simulink model "Requirements_Table"  (R2022b)
settings: Solver=FixedStepAuto  StartTime=0.0  StopTime=10.0  FixedStep=1e-3  RelTol=1e-3  EnableMultiTasking=on
settings Model: ExtModeTrigDuration=5  Creator=Ali Umar  LastModifiedBy=Ali Umar
settings OptimizationCC: EnhancedBackFolding=on  PassReuseOutputArgsAs=Individual arguments  ZeroExternalMemoryAtStartup=off  ZeroInternalMemoryAtStartup=off  MaxStackSize=64  OptimizeBlockOrder=speed  DifferentSizesBufferReuse=on  OptimizationCustomize=off  EfficientTunableParamExpr=on
settings DebuggingCC: ParameterTunabilityLossMsg=error
settings HardwareCC: ProdBitPerPointer=32  ProdBitPerSizeT=32  ProdBitPerPtrDiffT=32  ProdLargestAtomicInteger=Long  ProdLargestAtomicFloat=Double  ProdWordSize=32  ProdHWDeviceType=ARM Compatible->ARM Cortex
settings SFSimCC: MATLABDynamicMemAlloc=off
settings RTWCC: Description=Embedded Coder  SystemTargetFile=ert.tlc  HardwareBoard=NXP FRDM-K64F  TLCOptions="-aInlineSetEventsForThisBaseRateFcn=TLC_FALSE -aSuppressMultiTaskScheduler=TLC_FALSE  -aRateBasedStepFcn=0"  TemplateMakefile=ert_default_tmf  Toolchain=GNU Tools for ARM Embedded Processors
settings CodeAppCC: ForceParamTrailComments=on  IgnoreCustomStorageClasses=off  OperatorAnnotations=on  SimulinkDataObjDesc=on  SFDataObjDesc=on  InsertBlockDesc=on
settings ERTTargetCC: ExtModeTransport=4  ExtModeMexFile=sendToCommService

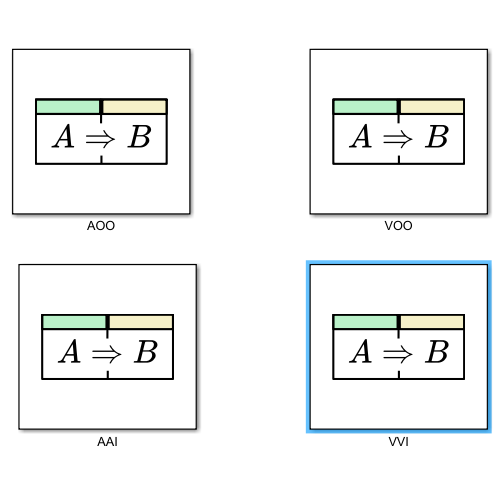
[thumbnail: Simulink's stored preview of the top-level diagram]
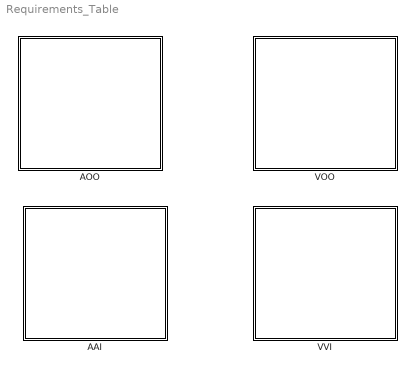
== system Requirements_Table ==
  AAI : Requirements Table  TreatAsAtomicUnit=on
  AOO : Requirements Table  TreatAsAtomicUnit=on
  VOO : Requirements Table  TreatAsAtomicUnit=on
  VVI : Requirements Table  TreatAsAtomicUnit=on

== stateflow chart Requirements_Table/VOO ==
  (default) -> (junction 1073741860)
  (junction 1073741860) -> (junction 1073741861) : {
      | % SF_REQ_REV_07
      | }
  (junction 1073741861) -> (junction 1073741863) : {
      | % HEADER_ASSIGNMENTS
      |
      | }
  (junction 1073741863) -> (junction 1073741865) : {
      | % START_A_4
      | }
  (junction 1073741865) -> (junction 1073741867) : {
      | }
  (junction 1073741867) -> (junction 1073741869)
  (junction 1073741869) -> (junction 1073741871) : {
      | }
  (junction 1073741871) -> (junction 1073741873) : {
      | % END_A_4
      | }
  (junction 1073741873) -> (junction 1073741976) : {
      | % START_R_1
      | }
  (junction 1073741976) -> (junction 1073741978) : {
      | }
  (junction 1073741978) -> (junction 1073741980)
  (junction 1073741980) -> (junction 1073741982) [order 1] : [duration((((ATR_PACE_CTRL) == (0))) && (((VENT_PACE_CTRL) == (1))) && (((PACE_CHARGE_CTRL) == (0))) && (((ATR_GND_CTRL) == (0))) && (((VENT_GND_CTRL) == (0)))) >= VPW]
  (junction 1073741980) -> (junction 1073741988) [order 2]
  (junction 1073741982) -> (junction 1073741984) : {
      | reqtable_postcondition((((ATR_PACE_CTRL) == (0))) && (((VENT_PACE_CTRL) == (0))) && (((PACING_REF_PWM) == (VA))) && (((PACE_CHARGE_CTRL) == (1))) && (((PACE_GND_CTRL) == (1))) && (((ATR_GND_CTRL) == (0))) && (((VENT_GND_CTRL) == (1))), 'R:1');
      | Charging C22 and Discharging C21
      |
      | }
  (junction 1073741984) -> (junction 1073741986) : {
      | }
  (junction 1073741986) -> (junction 1073741988)
  (junction 1073741988) -> (junction 1073741990)
  (junction 1073741990) -> (junction 1073741992) : {
      | % END_R_1
      | }
  (junction 1073741992) -> (junction 1073741955) : {
      | % START_R_7
      | }
  (junction 1073741955) -> (junction 1073741957) : {
      | }
  (junction 1073741957) -> (junction 1073741959)
  (junction 1073741959) -> (junction 1073741961) [order 1] : [duration((((ATR_PACE_CTRL) == (0))) && (((VENT_PACE_CTRL) == (0))) && (((PACING_REF_PWM) == (VA))) && (((PACE_CHARGE_CTRL) == (1))) && (((PACE_GND_CTRL) == (1))) && (((ATR_GND_CTRL) == (0))) && (((VENT_GND_CTRL) == (1)))) >= (60000/LRL)-VPW]
  (junction 1073741959) -> (junction 1073741967) [order 2]
  (junction 1073741961) -> (junction 1073741963) : {
      | reqtable_postcondition((((ATR_PACE_CTRL) == (0))) && (((VENT_PACE_CTRL) == (1))) && (((PACE_CHARGE_CTRL) == (0))) && (((ATR_GND_CTRL) == (0))) && (((VENT_GND_CTRL) == (0))), 'R:2');
      | VOO Pacing
      |
      | }
  (junction 1073741963) -> (junction 1073741965) : {
      | }
  (junction 1073741965) -> (junction 1073741967)
  (junction 1073741967) -> (junction 1073741969)
  (junction 1073741969) -> (junction 1073741971) : {
      | % END_R_7
      | }

== stateflow chart Requirements_Table/AAI ==
  (default) -> (junction 1073741860)
  (junction 1073741860) -> (junction 1073741861) : {
      | % SF_REQ_REV_07
      | }
  (junction 1073741861) -> (junction 1073741863) : {
      | % HEADER_ASSIGNMENTS
      |
      | }
  (junction 1073741863) -> (junction 1073741865) : {
      | % START_A_4
      | }
  (junction 1073741865) -> (junction 1073741867) : {
      | }
  (junction 1073741867) -> (junction 1073741869)
  (junction 1073741869) -> (junction 1073741871) : {
      | }
  (junction 1073741871) -> (junction 1073741873) : {
      | % END_A_4
      | }
  (junction 1073741873) -> (junction 1073742161) : {
      | % START_R_1
      | }
  (junction 1073742161) -> (junction 1073742163) : {
      | }
  (junction 1073742163) -> (junction 1073742165) : {
      | reqtable_postcondition((((FRONTEND_CTRL) == (1))) && (((ATR_CMP_REF_PWM) == (75))) && (((ATR_PACE_CTRL) == (0))) && (((VENT_PACE_CTRL) == (0))) && (((PACING_REF_PWM) == (75))) && (((PACE_CHARGE_CTRL) == (1))) && (((PACE_GND_CTRL) == (1))) && (((VENT_PACE_CTRL) == (0))) && (((ATR_PACE_CTRL) == (0))) && (((VENT_GND_CTRL) == (0))) && (((ATR_GND_CTRL) == (1))), 'R:1');
      | Startup Action
      |
      | }
  (junction 1073742165) -> (junction 1073742167) : {
      | }
  (junction 1073742167) -> (junction 1073741951) : {
      | % END_R_1
      | }
  (junction 1073741951) -> (junction 1073742194) : {
      | % START_R_22
      | }
  (junction 1073742194) -> (junction 1073742196) : {
      | }
  (junction 1073742196) -> (junction 1073742198)
  (junction 1073742198) -> (junction 1073742200) [order 1] : [duration((((FRONTEND_CTRL) == (1))) && (((ATR_CMP_REF_PWM) == (75))) && (((ATR_CMP_DETECT) == (0))) && (((ATR_PACE_CTRL) == (0))) && (((VENT_PACE_CTRL) == (0))) && (((PACING_REF_PWM) == (75))) && (((PACE_CHARGE_CTRL) == (1))) && (((PACE_GND_CTRL) == (1))) && (((VENT_PACE_CTRL) == (0))) && (((ATR_PACE_CTRL) == (0))) && (((VENT_GND_CTRL) == (0))) && (((ATR_GND_CTRL) == (1)))) >= LRI]
  (junction 1073742198) -> (junction 1073742206) [order 2]
  (junction 1073742200) -> (junction 1073742202) : {
      | reqtable_postcondition((((PACE_CHARGE_CTRL) == (0))) && (((PACE_GND_CTRL) == (1))) && (((VENT_PACE_CTRL) == (0))) && (((ATR_PACE_CTRL) == (1))) && (((VENT_GND_CTRL) == (0))) && (((ATR_GND_CTRL) == (0))), 'R:2');
      | pacing from the start
      |
      | }
  (junction 1073742202) -> (junction 1073742204) : {
      | }
  (junction 1073742204) -> (junction 1073742206)
  (junction 1073742206) -> (junction 1073742208)
  (junction 1073742208) -> (junction 1073742210) : {
      | % END_R_22
      | }
  (junction 1073742210) -> (junction 1073742173) : {
      | % START_R_16
      | }
  (junction 1073742173) -> (junction 1073742175) : {
      | }
  (junction 1073742175) -> (junction 1073742177)
  (junction 1073742177) -> (junction 1073742179) [order 1] : [duration((((FRONTEND_CTRL) == (1))) && (((ATR_CMP_REF_PWM) == (75))) && (((ATR_CMP_DETECT) == (0)))) >= LRI-R]
  (junction 1073742177) -> (junction 1073742185) [order 2]
  (junction 1073742179) -> (junction 1073742181) : {
      | reqtable_postcondition((((PACE_CHARGE_CTRL) == (0))) && (((PACE_GND_CTRL) == (1))) && (((VENT_PACE_CTRL) == (0))) && (((ATR_PACE_CTRL) == (1))) && (((VENT_GND_CTRL) == (0))) && (((ATR_GND_CTRL) == (0))), 'R:3');
      | Pacing
      |
      | }
  (junction 1073742181) -> (junction 1073742183) : {
      | }
  (junction 1073742183) -> (junction 1073742185)
  (junction 1073742185) -> (junction 1073742187)
  (junction 1073742187) -> (junction 1073742189) : {
      | % END_R_16
      | }
  (junction 1073742189) -> (junction 1073741967) : {
      | % START_R_10
      | }
  (junction 1073741967) -> (junction 1073741969) : {
      | }
  (junction 1073741969) -> (junction 1073741971)
  (junction 1073741971) -> (junction 1073741973) [order 1] : [duration((((FRONTEND_CTRL) == (1))) && (((ATR_CMP_REF_PWM) == (75))) && (((ATR_CMP_DETECT) == (1))) && (((ATR_PACE_CTRL) == (0))) && (((VENT_PACE_CTRL) == (0))) && (((PACING_REF_PWM) == (75))) && (((PACE_CHARGE_CTRL) == (1))) && (((PACE_GND_CTRL) == (1))) && (((VENT_PACE_CTRL) == (0))) && (((ATR_PACE_CTRL) == (0))) && (((VENT_GND_CTRL) == (0))) && (((ATR_GND_CTRL) == (1)))) >= LRI]
  (junction 1073741971) -> (junction 1073741979) [order 2]
  (junction 1073741973) -> (junction 1073741975) : {
      | reqtable_postcondition((((ATR_PACE_CTRL) == (0))) && (((VENT_PACE_CTRL) == (0))) && (((PACING_REF_PWM) == (75))) && (((PACE_CHARGE_CTRL) == (1))) && (((PACE_GND_CTRL) == (1))) && (((VENT_PACE_CTRL) == (0))) && (((ATR_PACE_CTRL) == (0))) && (((VENT_GND_CTRL) == (0))) && (((ATR_GND_CTRL) == (1))), 'R:4');
      | Timer checks refractory period and chargs C22/ Discharges C21
      |
      | }
  (junction 1073741975) -> (junction 1073741977) : {
      | }
  (junction 1073741977) -> (junction 1073741979)
  (junction 1073741979) -> (junction 1073741981)
  (junction 1073741981) -> (junction 1073741983) : {
      | % END_R_10
      | }
  (junction 1073741983) -> (junction 1073742000) : {
      | % START_R_13
      | }
  (junction 1073742000) -> (junction 1073742002) : {
      | }
  (junction 1073742002) -> (junction 1073742004)
  (junction 1073742004) -> (junction 1073742006) [order 1] : [duration((((ATR_CMP_DETECT) == (0))) && (((ATR_PACE_CTRL) == (0))) && (((VENT_PACE_CTRL) == (0))) && (((PACING_REF_PWM) == (75))) && (((PACE_CHARGE_CTRL) == (1))) && (((PACE_GND_CTRL) == (1))) && (((VENT_PACE_CTRL) == (0))) && (((ATR_PACE_CTRL) == (0))) && (((VENT_GND_CTRL) == (0))) && (((ATR_GND_CTRL) == (1)))) >= R]
  (junction 1073742004) -> (junction 1073742012) [order 2]
  (junction 1073742006) -> (junction 1073742008) : {
      | reqtable_postcondition((((FRONTEND_CTRL) == (1))) && (((ATR_CMP_REF_PWM) == (75))), 'R:5');
      | Turns sensing on
      |
      | }
  (junction 1073742008) -> (junction 1073742010) : {
      | }
  (junction 1073742010) -> (junction 1073742012)
  (junction 1073742012) -> (junction 1073742014)
  (junction 1073742014) -> (junction 1073742101) : {
      | % END_R_13
      | }

== stateflow chart Requirements_Table/AOO ==
  (default) -> (junction 1073741860)
  (junction 1073741860) -> (junction 1073741861) : {
      | % SF_REQ_REV_07
      | }
  (junction 1073741861) -> (junction 1073741863) : {
      | % HEADER_ASSIGNMENTS
      |
      | }
  (junction 1073741863) -> (junction 1073741865) : {
      | % START_A_4
      | }
  (junction 1073741865) -> (junction 1073741867) : {
      | }
  (junction 1073741867) -> (junction 1073741869)
  (junction 1073741869) -> (junction 1073741871) : {
      | }
  (junction 1073741871) -> (junction 1073741873) : {
      | % END_A_4
      | }
  (junction 1073741873) -> (junction 1073741996) : {
      | % START_R_1
      | }
  (junction 1073741996) -> (junction 1073741998) : {
      | }
  (junction 1073741998) -> (junction 1073742000)
  (junction 1073742000) -> (junction 1073742002) [order 1] : [duration((((ATR_PACE_CTRL) == (1))) && (((VENT_PACE_CTRL) == (0))) && (((PACE_CHARGE_CTRL) == (0))) && (((ATR_GND_CTRL) == (0))) && (((VENT_GND_CTRL) == (0)))) >= APW]
  (junction 1073742000) -> (junction 1073742008) [order 2]
  (junction 1073742002) -> (junction 1073742004) : {
      | reqtable_postcondition((((ATR_PACE_CTRL) == (0))) && (((VENT_PACE_CTRL) == (0))) && (((PACING_REF_PWM) == (AA))) && (((PACE_CHARGE_CTRL) == (1))) && (((PACE_GND_CTRL) == (1))) && (((ATR_GND_CTRL) == (1))) && (((VENT_GND_CTRL) == (0))), 'R:1');
      | Charges C22 Capacitor
      |
      | }
  (junction 1073742004) -> (junction 1073742006) : {
      | }
  (junction 1073742006) -> (junction 1073742008)
  (junction 1073742008) -> (junction 1073742010)
  (junction 1073742010) -> (junction 1073742012) : {
      | % END_R_1
      | }
  (junction 1073742012) -> (junction 1073742017) : {
      | % START_R_10
      | }
  (junction 1073742017) -> (junction 1073742019) : {
      | }
  (junction 1073742019) -> (junction 1073742021)
  (junction 1073742021) -> (junction 1073742023) [order 1] : [duration((((ATR_PACE_CTRL) == (0))) && (((VENT_PACE_CTRL) == (0))) && (((PACING_REF_PWM) == (AA))) && (((PACE_CHARGE_CTRL) == (1))) && (((PACE_GND_CTRL) == (1))) && (((ATR_GND_CTRL) == (1))) && (((VENT_GND_CTRL) == (0)))) >= (60000/LRL)-APW]
  (junction 1073742021) -> (junction 1073742029) [order 2]
  (junction 1073742023) -> (junction 1073742025) : {
      | reqtable_postcondition((((ATR_PACE_CTRL) == (1))) && (((VENT_PACE_CTRL) == (0))) && (((PACE_CHARGE_CTRL) == (0))) && (((ATR_GND_CTRL) == (0))) && (((VENT_GND_CTRL) == (0))), 'R:2');
      | AOO pacing
      |
      | }
  (junction 1073742025) -> (junction 1073742027) : {
      | }
  (junction 1073742027) -> (junction 1073742029)
  (junction 1073742029) -> (junction 1073742031)
  (junction 1073742031) -> (junction 1073742033) : {
      | % END_R_10
      | }

== stateflow chart Requirements_Table/VVI ==
  (default) -> (junction 1073741860)
  (junction 1073741860) -> (junction 1073741861) : {
      | % SF_REQ_REV_07
      | }
  (junction 1073741861) -> (junction 1073741863) : {
      | % HEADER_ASSIGNMENTS
      |
      | }
  (junction 1073741863) -> (junction 1073741865) : {
      | % START_A_4
      | }
  (junction 1073741865) -> (junction 1073741867) : {
      | }
  (junction 1073741867) -> (junction 1073741869)
  (junction 1073741869) -> (junction 1073741871) : {
      | }
  (junction 1073741871) -> (junction 1073741873) : {
      | % END_A_4
      | }
  (junction 1073741873) -> (junction 1073742161) : {
      | % START_R_1
      | }
  (junction 1073742161) -> (junction 1073742163) : {
      | }
  (junction 1073742163) -> (junction 1073742165) : {
      | reqtable_postcondition((((FRONTEND_CTRL) == (1))) && (((ATR_CMP_REF_PWM) == (75))) && (((ATR_PACE_CTRL) == (0))) && (((VENT_PACE_CTRL) == (0))) && (((PACING_REF_PWM) == (75))) && (((PACE_CHARGE_CTRL) == (1))) && (((PACE_GND_CTRL) == (1))) && (((VENT_PACE_CTRL) == (0))) && (((ATR_PACE_CTRL) == (0))) && (((VENT_GND_CTRL) == (1))) && (((ATR_GND_CTRL) == (0))), 'R:1');
      | Startup Action
      |
      | }
  (junction 1073742165) -> (junction 1073742167) : {
      | }
  (junction 1073742167) -> (junction 1073741951) : {
      | % END_R_1
      | }
  (junction 1073741951) -> (junction 1073742194) : {
      | % START_R_22
      | }
  (junction 1073742194) -> (junction 1073742196) : {
      | }
  (junction 1073742196) -> (junction 1073742198)
  (junction 1073742198) -> (junction 1073742200) [order 1] : [duration((((FRONTEND_CTRL) == (1))) && (((ATR_CMP_REF_PWM) == (75))) && (((ATR_CMP_DETECT) == (0))) && (((ATR_PACE_CTRL) == (0))) && (((VENT_PACE_CTRL) == (0))) && (((PACING_REF_PWM) == (75))) && (((PACE_CHARGE_CTRL) == (1))) && (((PACE_GND_CTRL) == (1))) && (((VENT_PACE_CTRL) == (0))) && (((ATR_PACE_CTRL) == (0))) && (((VENT_GND_CTRL) == (1))) && (((ATR_GND_CTRL) == (0)))) >= LRI]
  (junction 1073742198) -> (junction 1073742206) [order 2]
  (junction 1073742200) -> (junction 1073742202) : {
      | reqtable_postcondition((((PACE_CHARGE_CTRL) == (0))) && (((PACE_GND_CTRL) == (1))) && (((VENT_PACE_CTRL) == (1))) && (((ATR_PACE_CTRL) == (0))) && (((VENT_GND_CTRL) == (0))) && (((ATR_GND_CTRL) == (0))), 'R:2');
      | pacing from the start
      |
      | }
  (junction 1073742202) -> (junction 1073742204) : {
      | }
  (junction 1073742204) -> (junction 1073742206)
  (junction 1073742206) -> (junction 1073742208)
  (junction 1073742208) -> (junction 1073742210) : {
      | % END_R_22
      | }
  (junction 1073742210) -> (junction 1073742173) : {
      | % START_R_16
      | }
  (junction 1073742173) -> (junction 1073742175) : {
      | }
  (junction 1073742175) -> (junction 1073742177)
  (junction 1073742177) -> (junction 1073742179) [order 1] : [duration((((FRONTEND_CTRL) == (1))) && (((ATR_CMP_REF_PWM) == (75))) && (((ATR_CMP_DETECT) == (0)))) >= LRI-R]
  (junction 1073742177) -> (junction 1073742185) [order 2]
  (junction 1073742179) -> (junction 1073742181) : {
      | reqtable_postcondition((((PACE_CHARGE_CTRL) == (0))) && (((PACE_GND_CTRL) == (1))) && (((VENT_PACE_CTRL) == (1))) && (((ATR_PACE_CTRL) == (0))) && (((VENT_GND_CTRL) == (0))) && (((ATR_GND_CTRL) == (0))), 'R:3');
      | Pacing
      |
      | }
  (junction 1073742181) -> (junction 1073742183) : {
      | }
  (junction 1073742183) -> (junction 1073742185)
  (junction 1073742185) -> (junction 1073742187)
  (junction 1073742187) -> (junction 1073742189) : {
      | % END_R_16
      | }
  (junction 1073742189) -> (junction 1073741967) : {
      | % START_R_10
      | }
  (junction 1073741967) -> (junction 1073741969) : {
      | }
  (junction 1073741969) -> (junction 1073741971)
  (junction 1073741971) -> (junction 1073741973) [order 1] : [duration((((FRONTEND_CTRL) == (1))) && (((ATR_CMP_REF_PWM) == (75))) && (((ATR_CMP_DETECT) == (1))) && (((ATR_PACE_CTRL) == (0))) && (((VENT_PACE_CTRL) == (0))) && (((PACING_REF_PWM) == (75))) && (((PACE_CHARGE_CTRL) == (1))) && (((PACE_GND_CTRL) == (1))) && (((VENT_PACE_CTRL) == (0))) && (((ATR_PACE_CTRL) == (0))) && (((VENT_GND_CTRL) == (1))) && (((ATR_GND_CTRL) == (0)))) >= LRI]
  (junction 1073741971) -> (junction 1073741979) [order 2]
  (junction 1073741973) -> (junction 1073741975) : {
      | reqtable_postcondition((((ATR_PACE_CTRL) == (0))) && (((VENT_PACE_CTRL) == (0))) && (((PACING_REF_PWM) == (75))) && (((PACE_CHARGE_CTRL) == (1))) && (((PACE_GND_CTRL) == (1))) && (((VENT_PACE_CTRL) == (0))) && (((ATR_PACE_CTRL) == (0))) && (((VENT_GND_CTRL) == (1))) && (((ATR_GND_CTRL) == (0))), 'R:4');
      | Timer checks refractory period and chargs C22/ Discharges C21
      |
      | }
  (junction 1073741975) -> (junction 1073741977) : {
      | }
  (junction 1073741977) -> (junction 1073741979)
  (junction 1073741979) -> (junction 1073741981)
  (junction 1073741981) -> (junction 1073741983) : {
      | % END_R_10
      | }
  (junction 1073741983) -> (junction 1073742000) : {
      | % START_R_13
      | }
  (junction 1073742000) -> (junction 1073742002) : {
      | }
  (junction 1073742002) -> (junction 1073742004)
  (junction 1073742004) -> (junction 1073742006) [order 1] : [duration((((ATR_CMP_DETECT) == (0))) && (((ATR_PACE_CTRL) == (0))) && (((VENT_PACE_CTRL) == (0))) && (((PACING_REF_PWM) == (75))) && (((PACE_CHARGE_CTRL) == (1))) && (((PACE_GND_CTRL) == (1))) && (((VENT_PACE_CTRL) == (0))) && (((ATR_PACE_CTRL) == (0))) && (((VENT_GND_CTRL) == (1))) && (((ATR_GND_CTRL) == (0)))) >= R]
  (junction 1073742004) -> (junction 1073742012) [order 2]
  (junction 1073742006) -> (junction 1073742008) : {
      | reqtable_postcondition((((FRONTEND_CTRL) == (1))) && (((ATR_CMP_REF_PWM) == (75))), 'R:5');
      | Turns sensing on
      |
      | }
  (junction 1073742008) -> (junction 1073742010) : {
      | }
  (junction 1073742010) -> (junction 1073742012)
  (junction 1073742012) -> (junction 1073742014)
  (junction 1073742014) -> (junction 1073742101) : {
      | % END_R_13
      | }
